simulink model "PertControleAumentado"  (R2016b)
settings: Solver=ode45  StartTime=0.0  StopTime=700  RelTol=1e-3  EnableMultiTasking=on
settings Model: Creator=adolfobs  LastModifiedBy=adolfobs
settings DataIOCC: LimitDataPoints=on  MaxDataPoints=25000  SaveFormat=Array  SignalLoggingSaveFormat=ModelDataLogs
settings OptimizationCC: BlockReduction=off  BooleanDataType=off  InitFltsAndDblsToZero=on  LifeSpan=inf
settings DebuggingCC: SaveWithParameterizedLinksMsg=none  UnderspecifiedInitializationDetection=Classic  MergeDetectMultiDrivingBlocksExec=none  SignalResolutionControl=TryResolveAllWithWarning  MultiTaskDSMMsg=warning  MultiTaskCondExecSysMsg=none  SFUnexpectedBacktrackingDiag=warning  SFNoUnconditionalDefaultTransitionDiag=warning  SFExecutionAtInitializationDiag=none
settings HardwareCC: ProdBitPerPointer=32  ProdBitPerSizeT=32  ProdBitPerPtrDiffT=32  ProdLargestAtomicFloat=None  ProdIntDivRoundTo=Undefined  ProdEndianess=Unspecified  ProdWordSize=32  ProdHWDeviceType=32-bit Generic  TargetUnknown=on
settings ModelReferenceCC: PropagateSignalLabelsOutOfModel=off
settings GRTTargetCC: TargetFcnLib=ansi_tfl_tmw.mat  TargetLangStandard=C89/C90 (ANSI)  CombineOutputUpdateFcns=off  GRTInterface=on
settings ConfigComp: CovMetricSettings=dw  CovHtmlReporting=on  CovSaveCumulativeToWorkspaceVar=on  CovSaveSingleToWorkspaceVar=on  CovExternalEMLEnable=off

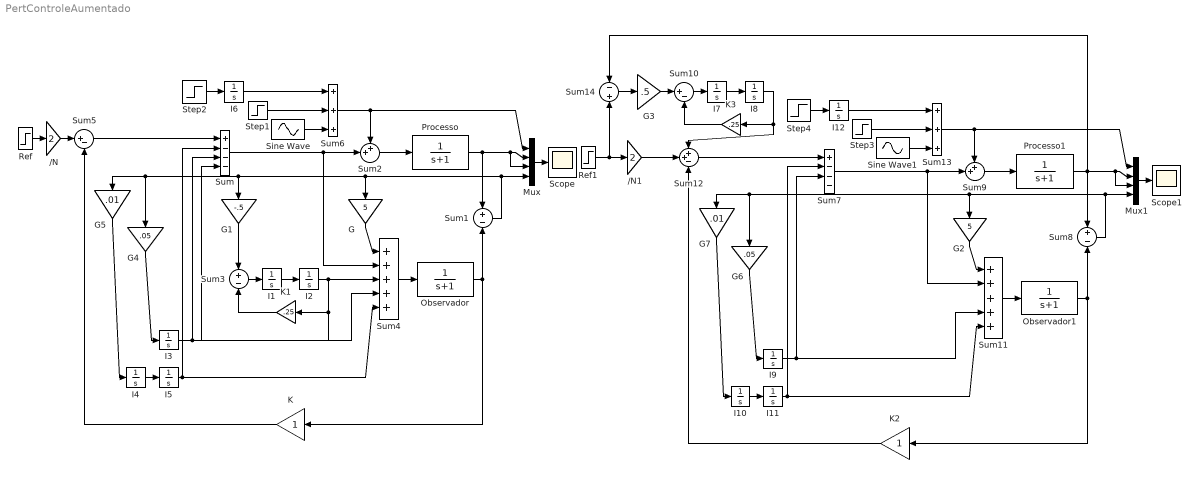
== system PertControleAumentado ==
  " /N" : Gain  Gain=2  SaturateOnIntegerOverflow=on  OutDataTypeStr=Inherit: Same as input  ParamDataTypeStr=Inherit: Same as input
  " /N1" : Gain  Gain=2  SaturateOnIntegerOverflow=on  OutDataTypeStr=Inherit: Same as input  ParamDataTypeStr=Inherit: Same as input
  G : Gain  Gain=5  SaturateOnIntegerOverflow=on  OutDataTypeStr=Inherit: Same as input  ParamDataTypeStr=Inherit: Same as input
  G1 : Gain  Gain=-.5  SaturateOnIntegerOverflow=on  OutDataTypeStr=Inherit: Same as input  ParamDataTypeStr=Inherit: Same as input
  G2 : Gain  Gain=5  SaturateOnIntegerOverflow=on  OutDataTypeStr=Inherit: Same as input  ParamDataTypeStr=Inherit: Same as input
  G3 : Gain  Gain=.5  SaturateOnIntegerOverflow=on  OutDataTypeStr=Inherit: Same as input  ParamDataTypeStr=Inherit: Same as input
  G4 : Gain  Gain=.05  SaturateOnIntegerOverflow=on  OutDataTypeStr=Inherit: Same as input  ParamDataTypeStr=Inherit: Same as input
  G5 : Gain  Gain=.01  SaturateOnIntegerOverflow=on  OutDataTypeStr=Inherit: Same as input  ParamDataTypeStr=Inherit: Same as input
  G6 : Gain  Gain=.05  SaturateOnIntegerOverflow=on  OutDataTypeStr=Inherit: Same as input  ParamDataTypeStr=Inherit: Same as input
  G7 : Gain  Gain=.01  SaturateOnIntegerOverflow=on  OutDataTypeStr=Inherit: Same as input  ParamDataTypeStr=Inherit: Same as input
  I{1..12} (12 alike) : Integrator
  K : Gain  SaturateOnIntegerOverflow=on  OutDataTypeStr=Inherit: Same as input  ParamDataTypeStr=Inherit: Same as input
  K1 : Gain  Gain=.25  SaturateOnIntegerOverflow=on  OutDataTypeStr=Inherit: Same as input  ParamDataTypeStr=Inherit: Same as input
  K2 : Gain  SaturateOnIntegerOverflow=on  OutDataTypeStr=Inherit: Same as input  ParamDataTypeStr=Inherit: Same as input
  K3 : Gain  Gain=.25  SaturateOnIntegerOverflow=on  OutDataTypeStr=Inherit: Same as input  ParamDataTypeStr=Inherit: Same as input
  Mux : Mux
  Mux1 : Mux
  Observador : TransferFcn  Denominator=[1 1]
  Observador1 : TransferFcn  Denominator=[1 1]
  Processo : TransferFcn  Denominator=[1 1]
  Processo1 : TransferFcn  Denominator=[1 1]
  Ref : Step  Time=100
  Ref1 : Step  Time=100
  Scope : Scope
  Scope1 : Scope
  Sine Wave : Sin  Amplitude=.3  Frequency=.5
  Sine Wave1 : Sin  Amplitude=.3  Frequency=.5
  Step1 : Step  Time=140  After=.2
  Step2 : Step  Time=400  After=.01
  Step3 : Step  Time=140  After=.2
  Step4 : Step  Time=400  After=.01
  Sum : Sum  Inputs=+---  SaturateOnIntegerOverflow=on  InputSameDT=on  OutDataTypeStr=Inherit: Same as first input
  Sum1 : Sum  Inputs=+-  SaturateOnIntegerOverflow=on  InputSameDT=on  OutDataTypeStr=Inherit: Same as first input
  Sum10 : Sum  Inputs=|+-  SaturateOnIntegerOverflow=on  InputSameDT=on  OutDataTypeStr=Inherit: Same as first input
  Sum11 : Sum  Inputs=+++++  SaturateOnIntegerOverflow=on  InputSameDT=on  OutDataTypeStr=Inherit: Same as first input
  Sum12 : Sum  Inputs=++-  SaturateOnIntegerOverflow=on  InputSameDT=on  OutDataTypeStr=Inherit: Same as first input
  Sum13 : Sum  Inputs=+++  SaturateOnIntegerOverflow=on  InputSameDT=on  OutDataTypeStr=Inherit: Same as first input
  Sum14 : Sum  Inputs=-+  SaturateOnIntegerOverflow=on  InputSameDT=on  OutDataTypeStr=Inherit: Same as first input
  Sum2 : Sum  Inputs=++|  SaturateOnIntegerOverflow=on  InputSameDT=on  OutDataTypeStr=Inherit: Same as first input
  Sum3 : Sum  Inputs=+|-  SaturateOnIntegerOverflow=on  InputSameDT=on  OutDataTypeStr=Inherit: Same as first input
  Sum4 : Sum  Inputs=+++++  SaturateOnIntegerOverflow=on  InputSameDT=on  OutDataTypeStr=Inherit: Same as first input
  Sum5 : Sum  Inputs=|+-  SaturateOnIntegerOverflow=on  InputSameDT=on  OutDataTypeStr=Inherit: Same as first input
  Sum6 : Sum  Inputs=+++  SaturateOnIntegerOverflow=on  InputSameDT=on  OutDataTypeStr=Inherit: Same as first input
  Sum7 : Sum  Inputs=+---  SaturateOnIntegerOverflow=on  InputSameDT=on  OutDataTypeStr=Inherit: Same as first input
  Sum8 : Sum  Inputs=+-  SaturateOnIntegerOverflow=on  InputSameDT=on  OutDataTypeStr=Inherit: Same as first input
  Sum9 : Sum  Inputs=++|  SaturateOnIntegerOverflow=on  InputSameDT=on  OutDataTypeStr=Inherit: Same as first input
  wires:
  Sum2/1 -> Processo/1
  Sum/1 -> Sum2/2, Sum4/2
  Mux/1 -> Scope/1
  Sum1/1 -> G/1, G1/1, G4/1, G5/1, Mux/4
  Sum3/1 -> I1/1
  I1/1 -> I2/1
  I2/1 -> Sum4/3, K1/1, Sum/4
  Observador/1 -> Sum1/2, K/1
  Sum4/1 -> Observador/1
  G/1 -> Sum4/1
  G1/1 -> Sum3/1
  Sum5/1 -> Sum/1
  K/1 -> Sum5/2
  Processo/1 -> Sum1/1, Mux/2, Mux/3
  Ref/1 -> " /N"/1
  " /N"/1 -> Sum5/1
  Sum6/1 -> Sum2/1, Mux/1
  I3/1 -> Sum4/4, Sum/3
  G4/1 -> I3/1
  G5/1 -> I4/1
  I4/1 -> I5/1
  I5/1 -> Sum/2, Sum4/5
  Sine Wave/1 -> Sum6/3
  Step1/1 -> Sum6/2
  Step2/1 -> I6/1
  I6/1 -> Sum6/1
  K1/1 -> Sum3/2
  Sum9/1 -> Processo1/1
  Sum7/1 -> Sum9/2, Sum11/2
  Mux1/1 -> Scope1/1
  Sum8/1 -> G2/1, G6/1, G7/1, Mux1/4
  Observador1/1 -> Sum8/2, K2/1
  Sum11/1 -> Observador1/1
  G2/1 -> Sum11/1
  Sum12/1 -> Sum7/1
  Processo1/1 -> Sum14/1, Sum8/1, Mux1/2, Mux1/3
  Ref1/1 -> Sum14/2, " /N1"/1
  Sum13/1 -> Sum9/1, Mux1/1
  I9/1 -> Sum11/4, Sum7/3
  G6/1 -> I9/1
  G7/1 -> I10/1
  I10/1 -> I11/1
  I11/1 -> Sum7/2, Sum11/5
  Sine Wave1/1 -> Sum13/3
  Step3/1 -> Sum13/2
  Step4/1 -> I12/1
  I12/1 -> Sum13/1
  Sum14/1 -> G3/1
  Sum10/1 -> I7/1
  I7/1 -> I8/1
  I8/1 -> Sum12/1, K3/1
  G3/1 -> Sum10/1
  K3/1 -> Sum10/2
  K2/1 -> Sum12/3
  " /N1"/1 -> Sum12/2
